simulink model "HW_1_2019a_final"  (R2020b)
settings: Solver=VariableStepAuto  StartTime=0.0  StopTime=70  RelTol=1e-12
model workspace (MAT data in the model file):
  d_tar = 20
values from neighbouring files (symbols this model uses):
  d_0 = 8    [acc1.m]
  d_m1 = 2    [acc1.m]
  d_m2 = 10    [acc1.m]
  t_H_tar = 1    [acc1.m]
  v_H0 = 28    [acc1.m]
  v_L0 = 36    [acc1.m]
  v_tar = 36    [acc1.m]
  x_H0 = 0    [acc1.m]
  x_L0 = 50    [acc1.m]
undefined symbols (not defined in the file or in its folder): sigbuilder_block
libraries: cstblocks x3, eeGeneralControl x1
settings Model: Creator=jake  LastModifiedBy=Iman
settings DebuggingCC: SFMachineParentedDataDiag=error
settings SFSimCC: CustomCodeUndefinedFunction=UseInterfaceOnly

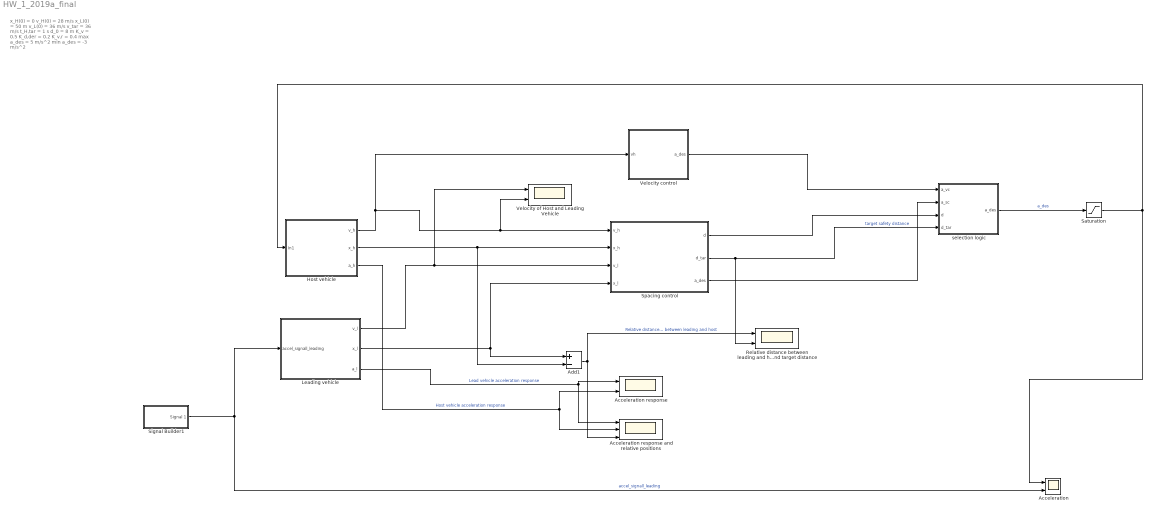
== system HW_1_2019a_final ==
  note: x_H(0) = 0
      | v_H(0) = 28 m/s
      |
      | x_L(0) = 50 m
      | v_L(0) = 36 m/s
      |
      | v_tar = 36 m/s
      | t_H,tar = 1 s
      | d_0 = 8 m
      |
      | K_v = 0.5
      | K_d,der = 0.2
      | K_v,r = 0.4
      |
      | max a_des = 5 m/s^2
      | min a_des = -3 m/s^2
  Acceleration : Scope  NumInputPorts=2
  Acceleration response : Scope  NumInputPorts=2
  Acceleration response and relative positions : Scope  NumInputPorts=3
  Add1 : Sum  Inputs=+-
  Host vehicle : Subsystem
  Leading vehicle : Subsystem
  Relative distance between leading and host and target distance : Scope  NumInputPorts=2
  Saturation : Saturate  UpperLimit=5  LowerLimit=-3
  Signal Builder1 : Subsystem  Tag=STV Subsys  LoadFcn=sigbuilder_block('load');  StartFcn=sigbuilder_block('start');  StopFcn=sigbuilder_block('stop');  ClipboardFcn=sigbuilder_block('clipboard');  mask(Sigbuilder block){tuvar=[0:10]}
      mask help: Simulink:masks:SigbuilderBlock_MD
      mask init:
      | if ~strcmp(get_param(bdroot(gcbh),'SimulationStatus'),'stopped') tuvar = sigbuilder_block('maskInit'); end
      settings: CopyFcn=sigbuilder_block('copy');  DeleteFcn=sigbuilder_block('delete');  ModelCloseFcn=sigbuilder_block('modelClose');  PreSaveFcn=sigbuilder_block('preSave');  PauseFcn=sigbuilder_block('pause');  ContinueFcn=sigbuilder_block('continue');  NameChangeFcn=sigbuilder_block('namechange');  OpenFcn=sigbuilder_block('open',[53.4 79.2 1033.2 459.6 ]);  CloseFcn=sigbuilder_block('close');
      mask Display: plot(0, 0, 100, 100,[2, 2, 32, 32, 2], [68, 8, 8, 68, 68],[32, 2], [38, 38], [32, 19, 2],[53, 60, 44], [32, 17, 17, 2],[16, 16, 31, 31]);txt = getActiveGroup(gcbh);text(2, 100, txt,'verticalAlignment', 'top');
  Spacing control : Subsystem
  Velocity control : Subsystem
  Velocity of Host and Leading Vehicle : Scope  NumInputPorts=2
  selection logic : Subsystem
  wires:
  selection logic/1(a_des) -> Saturation/1  "a_des"
  Signal Builder1/1(Signal 1) -> Leading vehicle/1(accel_signall_leading), Acceleration/2  "accel_signall_leading"
  Saturation/1 -> Acceleration/1, Host vehicle/1(In1)
  Host vehicle/1(v_h) -> Velocity control/1(vh), Velocity of Host and Leading Vehicle/2, Spacing control/1(v_h)
  Host vehicle/2(x_h) -> Add1/2, Spacing control/2(x_h)
  Leading vehicle/1(v_l) -> Velocity of Host and Leading Vehicle/1, Spacing control/3(v_l)
  Leading vehicle/2(x_l) -> Add1/1, Spacing control/4(x_l)
  Velocity control/1(a_des) -> selection logic/1(a_vc)
  Spacing control/3(a_des) -> selection logic/2(a_sc)
  Spacing control/1(d) -> selection logic/3(d)
  Spacing control/2(d_tar) -> Relative distance between leading and host and target distance/2, selection logic/4(d_tar)  "target safety distance"
  Add1/1 -> Relative distance between leading and host and target distance/1, Acceleration response and relative positions/3  "Relative distance between leading and host"
  Leading vehicle/3(a_l) -> Acceleration response and relative positions/1, Acceleration response/1  "Lead vehicle acceleration response"
  Host vehicle/3(a_h) -> Acceleration response and relative positions/2, Acceleration response/2  "Host vehicle acceleration response"

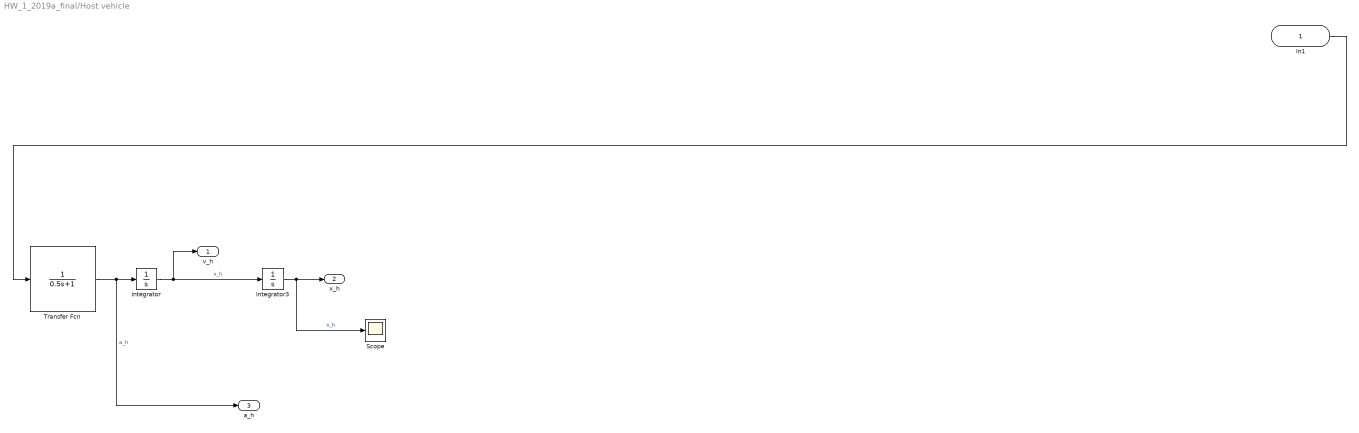
== system HW_1_2019a_final/Host vehicle ==
  In1 : Inport
  Integrator : Integrator  InitialCondition=v_H0
  Integrator3 : Integrator  InitialCondition=x_H0
  Scope : Scope
  Transfer Fcn : TransferFcn  Denominator=[0.5 1]
  v_h : Outport  VectorParamsAs1DForOutWhenUnconnected=off
  x_h : Outport  Port=2  VectorParamsAs1DForOutWhenUnconnected=off
  a_h : Outport  Port=3  VectorParamsAs1DForOutWhenUnconnected=off
  wires:
  Integrator/1 -> Integrator3/1, v_h/1  "v_h"
  Transfer Fcn/1 -> a_h/1, Integrator/1  "a_h"
  In1/1 -> Transfer Fcn/1
  Integrator3/1 -> Scope/1, x_h/1  "x_h"

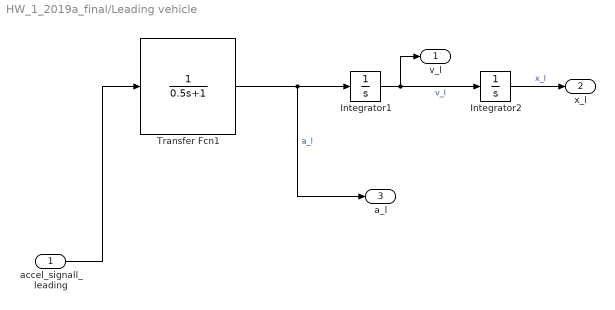
== system HW_1_2019a_final/Leading vehicle ==
  accel_signall_leading : Inport
  Integrator1 : Integrator  InitialCondition=v_L0
  Integrator2 : Integrator  InitialCondition=x_L0
  Transfer Fcn1 : TransferFcn  Denominator=[0.5 1]
  v_l : Outport  VectorParamsAs1DForOutWhenUnconnected=off
  x_l : Outport  Port=2  VectorParamsAs1DForOutWhenUnconnected=off
  a_l : Outport  Port=3  VectorParamsAs1DForOutWhenUnconnected=off
  wires:
  Integrator2/1 -> x_l/1  "x_l"
  accel_signall_leading/1 -> Transfer Fcn1/1
  Integrator1/1 -> Integrator2/1, v_l/1  "v_l"
  Transfer Fcn1/1 -> a_l/1, Integrator1/1  "a_l"

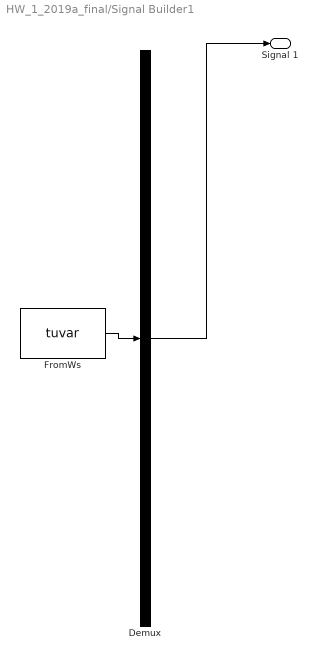
== system HW_1_2019a_final/Signal Builder1 ==
  Demux : Demux  Tag=STV Demux  Outputs=1
      settings: DisplayOption=none
  FromWs : FromWorkspace  Tag=STV FromWs  VariableName=tuvar
      SigBuilderData=|
      | common.afterFinalStr = 'Extrapolate'
      | common.sampleTime = 0
      | dataSet.timeRange = [0 46]
      | dataSet.name = 'Group 1'
      | sbobj.Groups.Name = 'Group 1'
      | sbobj.Groups.Signals.Name = 'Signal 1'
      | sbobj.Groups.Signals.XData = [0 10 10.5 13.5 14 40 40.5 43.5 44 46]
      | sbobj.Groups.Signals.YData = [0 0 -2 -2 0 0 2 2 0 0]
      | sbobj.Groups.TimeRange = [0 46]
  Signal 1 : Outport  Tag=STV Outport
  wires:
  Demux/1 -> Signal 1/1
  FromWs/1 -> Demux/1

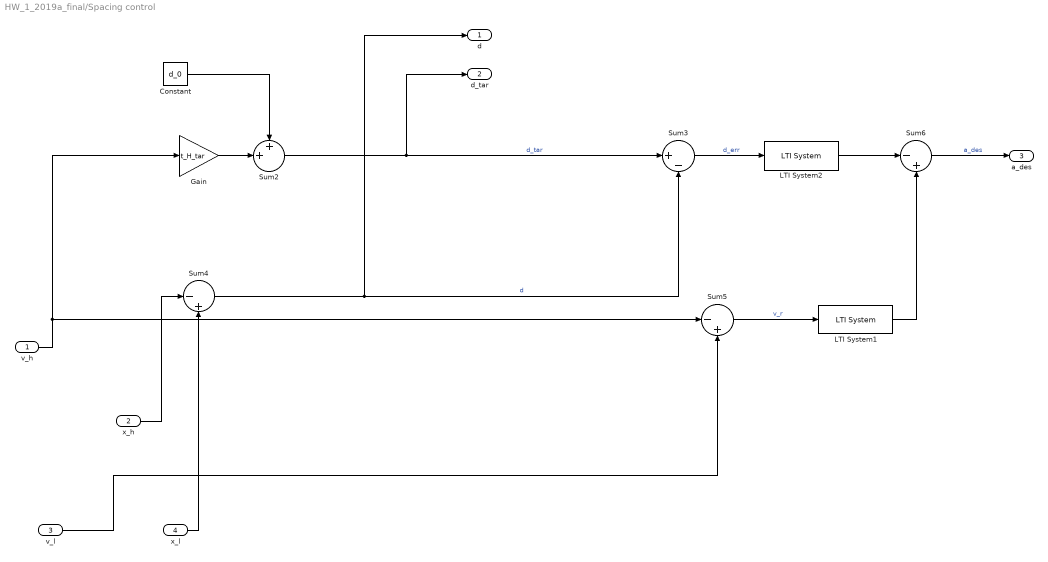
== system HW_1_2019a_final/Spacing control ==
  v_h : Inport
  x_h : Inport  Port=2
  v_l : Inport  Port=3
  x_l : Inport  Port=4
  Constant : Constant  Value=d_0
  Gain : Gain  Gain=t_H_tar
  LTI System1 : cstblocks/LTI System  sys=K_v_r  IC=[]
  LTI System2 : cstblocks/LTI System  sys=K_d_err  IC=[]
  Sum2 : Sum  Inputs=++|
  Sum3 : Sum  Inputs=|+-
  Sum4 : Sum  Inputs=|-+
  Sum5 : Sum  Inputs=|-+
  Sum6 : Sum  Inputs=|-+
  d : Outport  VectorParamsAs1DForOutWhenUnconnected=off
  d_tar : Outport  Port=2  VectorParamsAs1DForOutWhenUnconnected=off
  a_des : Outport  Port=3  VectorParamsAs1DForOutWhenUnconnected=off
  wires:
  x_l/1 -> Sum4/2
  v_l/1 -> Sum5/2
  Sum6/1 -> a_des/1  "a_des"
  Sum4/1 -> d/1, Sum3/2  "d"
  LTI System1/1 -> Sum6/2
  v_h/1 -> Sum5/1, Gain/1
  Gain/1 -> Sum2/2
  Sum5/1 -> LTI System1/1  "v_r"
  Sum3/1 -> LTI System2/1  "d_err"
  x_h/1 -> Sum4/1
  Sum2/1 -> d_tar/1, Sum3/1  "d_tar"
  Constant/1 -> Sum2/1
  LTI System2/1 -> Sum6/1

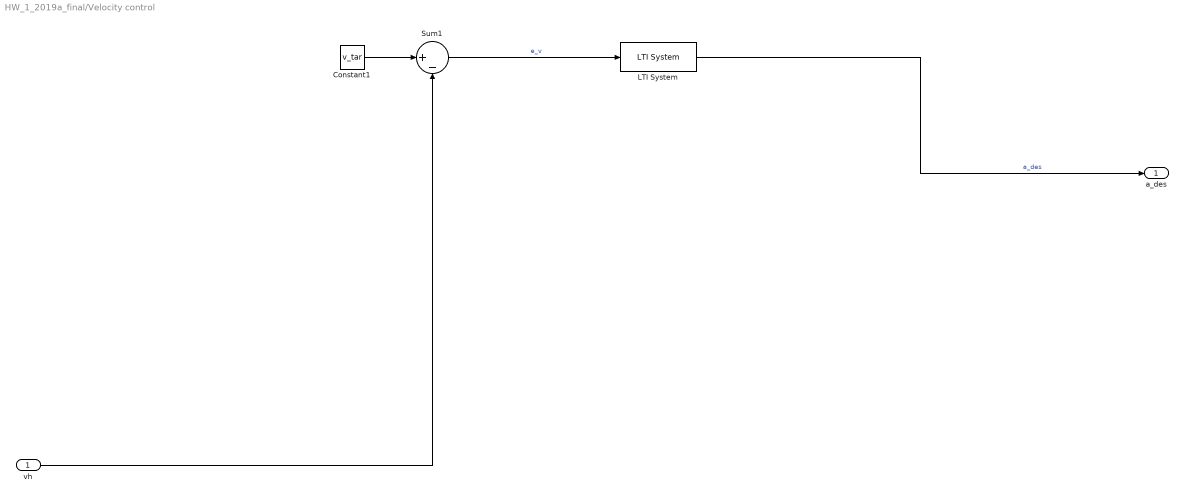
== system HW_1_2019a_final/Velocity control ==
  vh : Inport
  Constant1 : Constant  Value=v_tar
  LTI System : cstblocks/LTI System  sys=K_v  IC=[]
  Sum1 : Sum  Inputs=|+-
  a_des : Outport  VectorParamsAs1DForOutWhenUnconnected=off
  wires:
  LTI System/1 -> a_des/1  "a_des"
  vh/1 -> Sum1/2
  Constant1/1 -> Sum1/1
  Sum1/1 -> LTI System/1  "e_v"

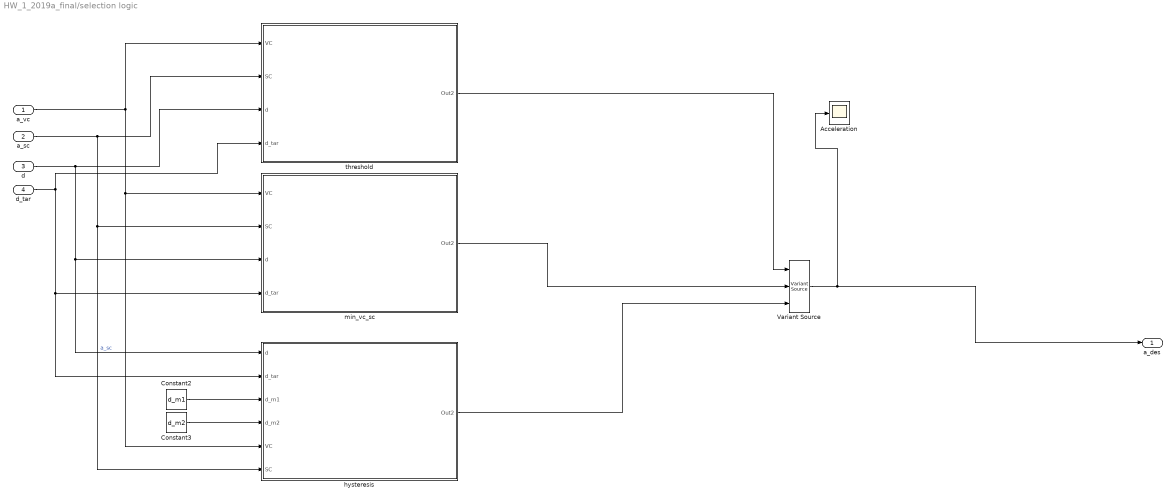
== system HW_1_2019a_final/selection logic ==
  a_vc : Inport
  a_sc : Inport  Port=2
  d : Inport  Port=3
  d_tar : Inport  Port=4
  Acceleration : Scope
  Constant2 : Constant  Value=d_m1
  Constant3 : Constant  Value=d_m2
  Variant Source : VariantSource
  hysteresis : Subsystem
  min_vc_sc : Subsystem
  threshold : Subsystem
  a_des : Outport  VectorParamsAs1DForOutWhenUnconnected=off
  wires:
  a_sc/1 -> hysteresis/6(SC), min_vc_sc/2(SC), threshold/2(SC)  "a_sc"
  a_vc/1 -> threshold/1(VC), hysteresis/5(VC), min_vc_sc/1(VC)
  Constant2/1 -> hysteresis/3(d_m1)
  Constant3/1 -> hysteresis/4(d_m2)
  hysteresis/1(Out2) -> Variant Source/3
  d/1 -> threshold/3(d), hysteresis/1(d), min_vc_sc/3(d)
  d_tar/1 -> hysteresis/2(d_tar), min_vc_sc/4(d_tar), threshold/4(d_tar)
  min_vc_sc/1(Out2) -> Variant Source/2
  threshold/1(Out2) -> Variant Source/1
  Variant Source/1 -> Acceleration/1, a_des/1

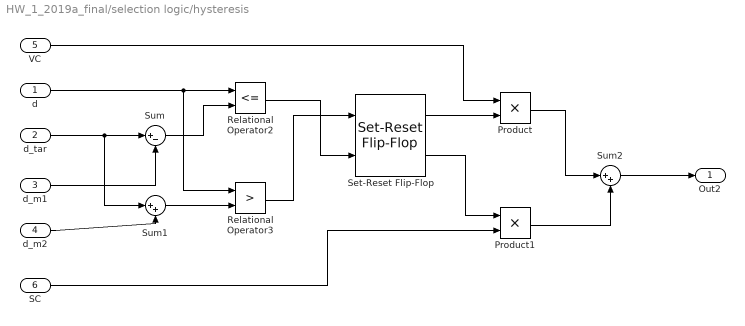
== system HW_1_2019a_final/selection logic/hysteresis ==
  d : Inport
  d_tar : Inport  Port=2
  d_m1 : Inport  Port=3
  d_m2 : Inport  Port=4
  VC : Inport  Port=5
  SC : Inport  Port=6
  Product : Product
  Product1 : Product
  Relational Operator2 : RelationalOperator  Operator=<=  OutDataTypeStr=boolean  RndMeth=Simplest
  Relational Operator3 : RelationalOperator  Operator=>  OutDataTypeStr=boolean  RndMeth=Simplest
  Set-Reset Flip-Flop : eeGeneralControl/Set-Reset Flip-Flop  LabelModeActiveChoice=Discrete  UndefState=Set  Q0=0  Ts=-1
      settings: SourceProductBaseCode=PS
  Sum : Sum  Inputs=|+-
  Sum1 : Sum  Inputs=|++
  Sum2 : Sum  Inputs=|++
  Out2 : Outport
  wires:
  d_m2/1 -> Sum1/2
  Sum1/1 -> Relational Operator3/2
  Relational Operator2/1 -> Set-Reset Flip-Flop/2
  VC/1 -> Product/1
  SC/1 -> Product1/2
  Relational Operator3/1 -> Set-Reset Flip-Flop/1
  Sum/1 -> Relational Operator2/2
  d_m1/1 -> Sum/2
  d/1 -> Relational Operator3/1, Relational Operator2/1
  d_tar/1 -> Sum1/1, Sum/1
  Product1/1 -> Sum2/2
  Product/1 -> Sum2/1
  Sum2/1 -> Out2/1
  Set-Reset Flip-Flop/1 -> Product/2
  Set-Reset Flip-Flop/2 -> Product1/1

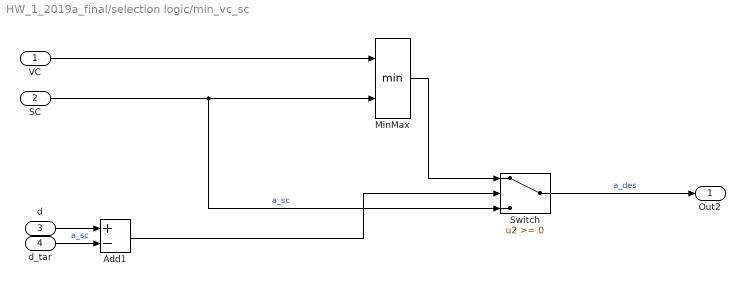
== system HW_1_2019a_final/selection logic/min_vc_sc ==
  VC : Inport
  SC : Inport  Port=2
  d : Inport  Port=3
  d_tar : Inport  Port=4
  Add1 : Sum  Inputs=+-
  MinMax : MinMax  Inputs=2
  Switch : Switch
  Out2 : Outport
  wires:
  Add1/1 -> Switch/2
  MinMax/1 -> Switch/1
  VC/1 -> MinMax/1
  SC/1 -> Switch/3, MinMax/2  "a_sc"
  Switch/1 -> Out2/1  "a_des"
  d/1 -> Add1/1
  d_tar/1 -> Add1/2  "a_sc"

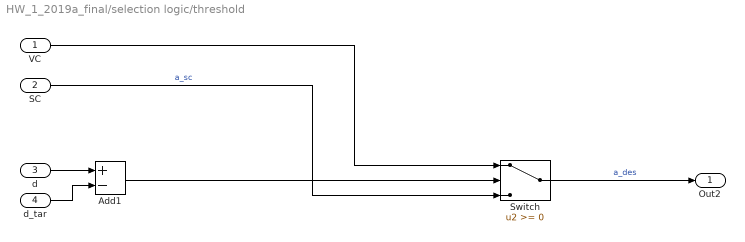
== system HW_1_2019a_final/selection logic/threshold ==
  VC : Inport
  SC : Inport  Port=2
  d : Inport  Port=3
  d_tar : Inport  Port=4
  Add1 : Sum  Inputs=+-
  Switch : Switch
  Out2 : Outport
  wires:
  Add1/1 -> Switch/2
  SC/1 -> Switch/3  "a_sc"
  Switch/1 -> Out2/1  "a_des"
  d/1 -> Add1/1
  d_tar/1 -> Add1/2
  VC/1 -> Switch/1
